simulink library "mylib"  (R2021a)
settings: Solver=VariableStepAuto  StartTime=0.0  StopTime=10.0  RelTol=1e-3
settings Model: Creator=Aula  LastModifiedBy=Aula

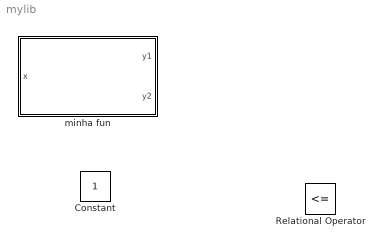
== system mylib ==
  Constant : Constant
  Relational Operator : RelationalOperator  Operator=<=  OutDataTypeStr=boolean  RndMeth=Simplest
  minha fun : Subsystem  mask(Função Matematica){k=2}
      mask prompts: k "Ganho (k)"
      mask help: Essa função faz uma operação matematica
      mask init:
      | if k > 10
      |     c = 1;
      | else
      |     c = -1;
      | end
      mask Help:
      | Essa função faz uma operação matematica tem esses parametros
      | 
      | ganho k
      | uma constante c
      mask Display:
      | disp('y_1 = k*x^2; y_2 = c');
      | port_label('input', 1, 'x');
      | port_label('output', 1, 'y1');
      | port_label('output', 2, 'y2');

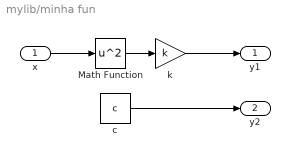
== system mylib/minha fun ==
  x : Inport
  Math Function : Math  Operator=square  SaturateOnIntegerOverflow=on
  c : Constant  Value=c
  k : Gain  Gain=k
  y1 : Outport
  y2 : Outport  Port=2
  wires:
  x/1 -> Math Function/1
  Math Function/1 -> k/1
  c/1 -> y2/1
  k/1 -> y1/1
